simulink model "test_calibrate"  (R2018a)
settings: Solver=FixedStepDiscrete  StartTime=0.0  StopTime=inf  FixedStep=0.010  RelTol=1e-3  EnableMultiTasking=on
libraries: arduinolib x2, dspstat3 x2
settings Model: SimulationMode=external  ExtModeTrigDuration=2  Creator=Gergely  LastModifiedBy=Gergely
settings OptimizationCC: EnhancedBackFolding=on  PassReuseOutputArgsAs=Individual arguments  MaxStackSize=64  OptimizeBlockOrder=speed  DifferentSizesBufferReuse=on  OptimizationCustomize=off
settings DebuggingCC: ParameterTunabilityLossMsg=error
settings HardwareCC: ProdBitPerInt=16  ProdBitPerPointer=16  ProdBitPerSizeT=16  ProdBitPerPtrDiffT=16  ProdLargestAtomicFloat=None  ProdWordSize=8  ProdHWDeviceType=Atmel->AVR
settings SFSimCC: MATLABDynamicMemAlloc=off
settings RTWCC: SystemTargetFile=ert.tlc  HardwareBoard=Arduino Uno  TLCOptions=-aInlineSetEventsForThisBaseRateFcn=TLC_FALSE -aSuppressMultiTaskScheduler=TLC_FALSE -aRateBasedStepFcn=1  TemplateMakefile=ert_default_tmf  GenerateReport=on  Toolchain=Arduino AVR  BuildConfiguration=Faster Runs  IncludeHyperlinkInReport=on  LaunchReport=on  GenerateTraceInfo=on  GenerateTraceReport=on  GenerateTraceReportSl=on  GenerateTraceReportSf=on  GenerateTraceReportEml=on
settings CodeAppCC: ForceParamTrailComments=on  IgnoreCustomStorageClasses=off  OperatorAnnotations=on  SimulinkDataObjDesc=on  SFDataObjDesc=on  InsertBlockDesc=on
settings ERTTargetCC: SupportContinuousTime=on  SupportVariableSizeSignals=on

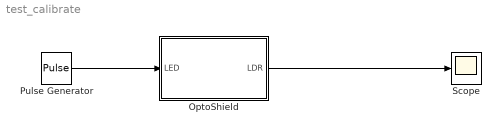
== system test_calibrate ==
  OptoShield : Subsystem
      mask Display: image('C:\Dropbox\_school_\_research_\__AutomationShield__\__GIT__\Gergely\AutomationShield\simulink\icons\test.svg');
  Pulse Generator : DiscretePulseGenerator  PulseType=Time based  Amplitude=60  Period=2.1  PulseWidth=50
  Scope : Scope
  wires:
  Pulse Generator/1 -> OptoShield/1(LED)
  OptoShield/1(LDR) -> Scope/1

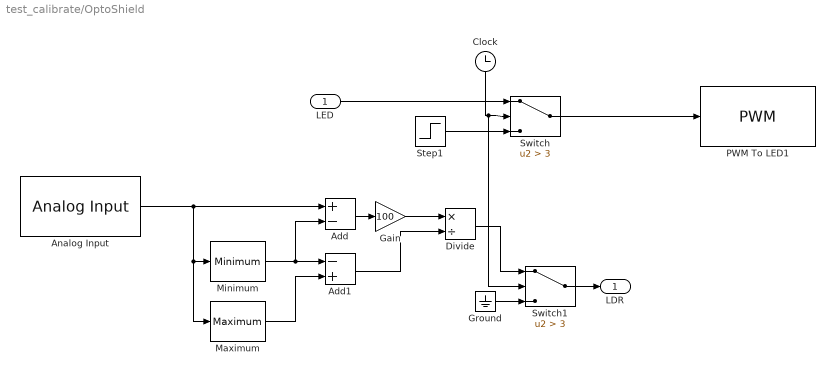
== system test_calibrate/OptoShield ==
  LED : Inport
  Add : Sum  Inputs=+-
  Add1 : Sum  Inputs=-+
  Analog Input : arduinolib/Analog Input  pinNumber=1  ReadResultsOnly=off  ConversionTriggerSource=Software  ExternalTriggerType=uint32(0)  OutputDataType=uint16  EnableConversionCompleteNotify=off  EnableOuputStatus=off  SampleTime=0.01  blockPlatform=arduino
  Clock : Clock
  Divide : Product  Inputs=*/
  Gain : Gain  Gain=100
  Ground : Ground
  Maximum : dspstat3/Maximum  operation=maximum  fcn=Running  indexBase=One  operateOver=Each column  Dimension=1  InputProcessing=Columns as channels (frame based)  reset=None  roiEnable=off  roiType=Rectangles  roiPortion=Entire ROI  roiOutput=Individual statistics for each ROI  roiFlag=off  roundingMode=Floor  overflowMode=off  accumDataTypeStr=Inherit: Same as product output  accumLastDataTypeStr=Inherit: Same as product output
  Minimum : dspstat3/Minimum  operation=minimum  fcn=Running  indexBase=One  operateOver=Each column  Dimension=1  InputProcessing=Columns as channels (frame based)  reset=None  roiEnable=off  roiType=Rectangles  roiPortion=Entire ROI  roiOutput=Individual statistics for each ROI  roiFlag=off  roundingMode=Floor  overflowMode=off
      settings: SourceProductName=DSP System Toolbox  SourceProductBaseCode=DS
  PWM To LED1 : arduinolib/PWM  pinNumber=3  EnableInputFrequency=off  InitialFrequency=2000  InitialDutyCycle=0  NotificationType=None  blockPlatform=arduino
  Step1 : Step  Time=1.5  After=255  SampleTime=0.010
  Switch : Switch  Criteria=u2 > Threshold  Threshold=3
  Switch1 : Switch  Criteria=u2 > Threshold  Threshold=3
  LDR : Outport
  wires:
  Minimum/1 -> Add1/1, Add/2
  Maximum/1 -> Add1/2
  Clock/1 -> Switch/2, Switch1/2
  LED/1 -> Switch/1
  Add/1 -> Gain/1
  Add1/1 -> Divide/2
  Gain/1 -> Divide/1
  Switch/1 -> PWM To LED1/1
  Analog Input/1 -> Minimum/1, Maximum/1, Add/1
  Step1/1 -> Switch/3
  Divide/1 -> Switch1/1
  Ground/1 -> Switch1/3
  Switch1/1 -> LDR/1
